simulink model "Boost"  (R2018b)
settings: Solver=ode15s  StartTime=0.0  StopTime=2e-3  RelTol=1e-4  EnableMultiTasking=on
settings Model: Creator=Tran Minh  LastModifiedBy=UngBK
settings DataIOCC: LimitDataPoints=on  SaveFormat=Array
settings OptimizationCC: LifeSpan=inf
settings DebuggingCC: SolverPrmCheckMsg=warning  LibraryContextMissingDiagnostic=none  SFUnexpectedBacktrackingDiag=warning  SFNoUnconditionalDefaultTransitionDiag=warning  SFExecutionAtInitializationDiag=none
settings HardwareCC: ProdBitPerPointer=32  ProdBitPerSizeT=32  ProdBitPerPtrDiffT=32  ProdLargestAtomicFloat=None  ProdIntDivRoundTo=Undefined  ProdEndianess=Unspecified  ProdWordSize=32  ProdHWDeviceType=32-bit Generic
settings ModelReferenceCC: PropagateSignalLabelsOutOfModel=off
settings SFSimCC: SimUseLocalCustomCode=off
settings RTWCC: RTWUseLocalCustomCode=off
settings CodeAppCC: StateflowObjectComments=on
settings GRTTargetCC: TargetLangStandard=C89/C90 (ANSI)  GeneratePreprocessorConditionals=Disable all
settings ConfigComp: CovMetricSettings=dw  CovHtmlReporting=on  CovSaveCumulativeToWorkspaceVar=on  CovSaveSingleToWorkspaceVar=on  CovExternalEMLEnable=off  CovSFcnEnable=off

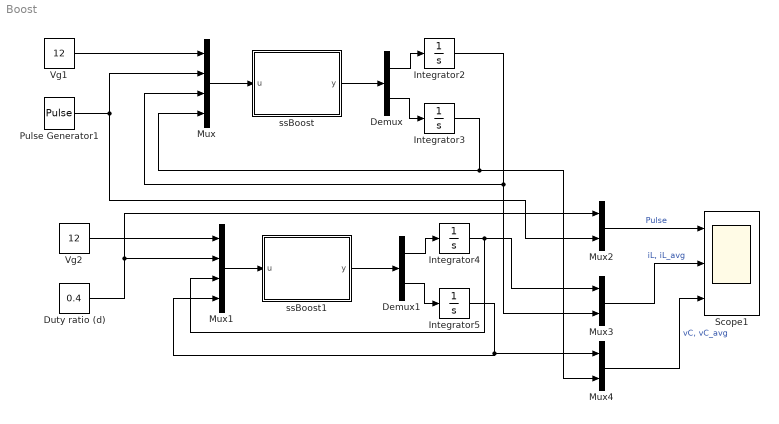
== system Boost ==
  Demux : Demux  Outputs=2
  Demux1 : Demux  Outputs=2
  Duty ratio (d) : Constant  Value=0.4
  Integrator{2..5} (4 alike) : Integrator
  Mux : Mux
  Mux1 : Mux
  Mux2 : Mux  Inputs=2
  Mux3 : Mux  Inputs=2
  Mux4 : Mux  Inputs=2
  Pulse Generator1 : DiscretePulseGenerator  PulseType=Time based  Period=1/50e3  PulseWidth=40
  Scope1 : Scope  NumInputPorts=3
  Vg1 : Constant  Value=12
  Vg2 : Constant  Value=12
  ssBoost : MATLAB Function  TreatAsAtomicUnit=on
  ssBoost1 : MATLAB Function  TreatAsAtomicUnit=on
  wires:
  Mux/1 -> ssBoost/1(u)
  ssBoost/1(y) -> Demux/1
  Demux/1 -> Integrator2/1
  Demux/2 -> Integrator3/1
  Integrator3/1 -> Mux4/2, Mux/4
  Vg1/1 -> Mux/1
  Mux1/1 -> ssBoost1/1(u)
  ssBoost1/1(y) -> Demux1/1
  Demux1/1 -> Integrator4/1
  Demux1/2 -> Integrator5/1
  Integrator5/1 -> Mux1/4, Mux4/1
  Integrator4/1 -> Mux1/3, Mux3/1
  Duty ratio (d)/1 -> Mux1/2, Mux2/1
  Vg2/1 -> Mux1/1
  Pulse Generator1/1 -> Mux2/2, Mux/2
  Integrator2/1 -> Mux3/2, Mux/3
  Mux2/1 -> Scope1/1  "Pulse"
  Mux3/1 -> Scope1/2  "iL, iL_avg"
  Mux4/1 -> Scope1/3  "vC, vC_avg"

== matlab function Boost/ssBoost1 ==
  data: u input size=4; y output
function y = ssBoost(u)
%#codegen
%Constants
L=480e-6;
C=40e-6;
R=10;

%inputs
Vg=u(1);
d=u(2);
iL=u(3);
vC=u(4);
%%%%
diL=(Vg-vC*(1-d))/L;
diC =(iL*(1-d)-vC/R)/C;

y = [diL diC];

== matlab function Boost/ssBoost ==
  data: u input size=4; y output
function y = ssBoost(u)
%#codegen
%Constants
L=480e-6;
C=40e-6;
R=10;

%inputs
Vg=u(1);
d=u(2);
iL=u(3);
vC=u(4);
%%%%
diL=(Vg-vC*(1-d))/L;
diC =(iL*(1-d)-vC/R)/C;

y = [diL diC];
